simulink model "aa_IOT"  (R2024b)
settings: Solver=VariableStepAuto  StartTime=0.0  StopTime=0.20  RelTol=1e-3
undefined symbols (not defined in the file): Acid, Ion, Lead, Lithium, sigbuilder_block
libraries: spsBreakerLib x120, spsBatteryLib x72, spsSeriesRLCBranchLib x47, spsVoltageMeasurementLib x33, spsIdealSwitchLib x19, spsDiodeLib x10, spsCurrentMeasurementLib x8, spsThyristorLib x6, sldrtlib x4, spsACVoltageSourceLib x3, spsIGBTLib x2, spsPVArrayLib x1
(part 1 of 7)
settings Model: SimulationMode=accelerator  Creator=Jatay  LastModifiedBy=Jatay

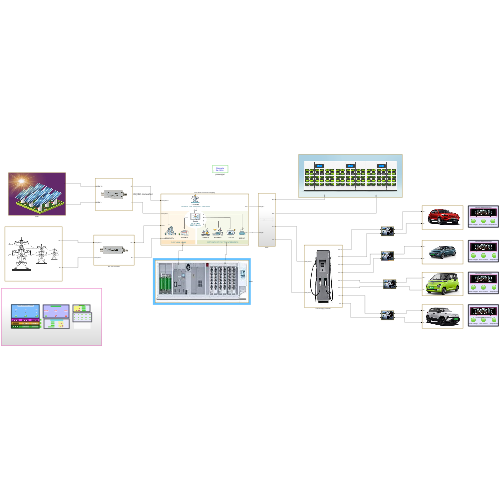
[thumbnail: Simulink's stored preview of the top-level diagram]
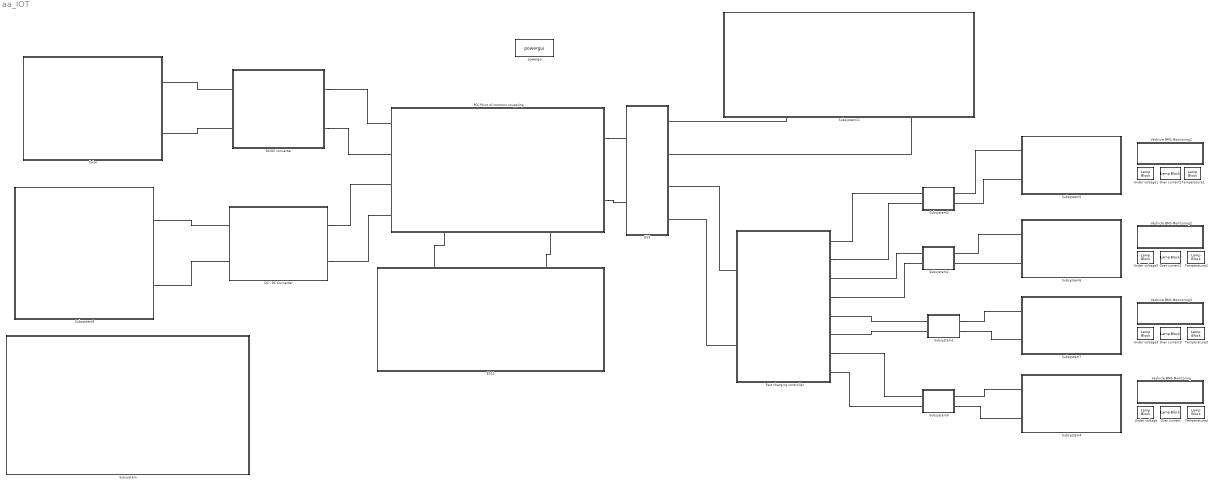
== system aa_IOT ==
  DC - DC Converter : Subsystem
      mask Display: image('cc_converter.png');
  DC/DC converter : Subsystem
      mask Display: image('cc_converter.png');
  ESS : Subsystem
  ESS1 : Subsystem
      mask Display: image('ess.jpeg');
  Fast charging controller : Subsystem
      mask Display: image('FC.jpeg');
  Over current{,1..3} (4 alike) : LampBlock  LabelPosition=Hide
  PCC Point of common couppling : Subsystem
      settings: PortSchema="{\"entries\":[{\"content\":{\"sides\":[{\"content\":{\"connectorIds\":[\"LConn1\",\"LConn2\",\"LConn3\",\"LConn4\"]},\"type\":\"ConnectorPlacement.EquallySpacedRectSide\",\"uuid\":\"0b8ed45c-57e4-41e0-bfb2-9585222a0f80\"},{\"content\":{\"connectorIds\":[\"RConn1\",\"RConn2\"],\"side\":\"RIGHT\"},\"type\":\"ConnectorPlacement.EquallySpacedRectSide\",\"uuid\":\"94498682-9e53-424b-ae3f-72f463f0ef3d\"},{\"content\":{\"side\":\"TOP\"},\"type\":\"ConnectorPlacement.EquallySpacedRectSide\",\"uuid\":\"67a2b653-7e16-402f-9cd2-3c5333b5ea45\"},{\"content\":{\"connectorIds\":[\"RConn3\",\"RConn4\"],\"side\":\"BOTTOM\"},\"type\":\"ConnectorPlacement.EquallySpacedRectSide\",\"uuid\":\"cc71de87-45eb-4874-8a05-0c8232189766\"}]},\"type\":\"ConnectorPlacement.EquallySpacedConnector\",\"uuid\":\"bd8a6289-7e4b-491d-b567-63bc7d53a2fa\"}],\"packageUris\":[\"http://schema.mathworks.com/mf0/Connector/R2020b\"],\"version\":\"1.0\"}"
      mask Display: image('pcc.png');
  Solar : Subsystem
      mask Display: image('Solar-Power-Plant-1024x536.jpg');
  Subsystem : Subsystem
  Subsystem1 : Subsystem
      mask Display: image('plugin.jpeg');
  Subsystem11 : Subsystem
      mask Display: image('swapping.webp');
  Subsystem2 : Subsystem
      mask Display: image('plugin.jpeg');
  Subsystem3 : Subsystem
      mask Display: image('plugin.jpeg');
  Subsystem4 : Subsystem
      mask Display: image('ev_4.webp');
  Subsystem5 : Subsystem
      mask Display: image('ev_3.webp');
  Subsystem6 : Subsystem
      mask Display: image('ev_2.jpg');
  Subsystem7 : Subsystem
      mask Display: image('ev-1.jpeg');
  Subsystem8 : Subsystem
      mask Display: image('grid.png');
  Subsystem9 : Subsystem
      mask Display: image('plugin.jpeg');
  Temperature{1..4} (4 alike) : LampBlock  LabelPosition=Hide
  Under voltage{,1..3} (4 alike) : LampBlock  LabelPosition=Hide
  Vechicle BMS Monitoring : Subsystem
      mask Display: image('Dash_board.jpeg');
  Vechicle BMS Monitoring1 : Subsystem
      mask Display: image('Dash_board.jpeg');
  Vechicle BMS Monitoring2 : Subsystem
      mask Display: image('Dash_board.jpeg');
  Vechicle BMS Monitoring3 : Subsystem
      mask Display: image('Dash_board.jpeg');
  powergui : sps_lib/powergui  Priority=1  SimulationMode=Discrete  SampleTime=5e-6  frequency=60  Iterations=50  frequencyindice=0  Pbase=100e6  ErrMax=1e-4  UnitsV=kV  UnitsW=MW  buscounter=0  FunctionMessages=off  echomessages=off  EnableUseOfTLC=off  CurrentSourceSwitches=off  DisableSnubberDevices=off  DisableRonSwitches=off  DisableVfSwitches=off  DisplayEquations=off  AutomaticDiscreteSolvers=off  SolverType=Tustin  Interpol=off  ExternalGateDelay=off  methode=off  Ts=0  x0status=blocks  SPID=off  SwTol=0  HookPort=off  NonlinearTolerance=1e-4  nMaxIteration=100  ContinueOnMaxIteration=off  RestoreLinks=warning  ResistiveCurrentMeasurement=off  Frange=[0:2:500]  Ylog=off  Xlog=on  ShowGrid=off  save=off  variable=ZData  structure=0  ZoomFFT=off  StartTime=0.0  cycles=1  DisplayStyle=1  fundamental=60  FreqAxis=off  MaxFrequency=1000  frequencyindicesteady=1  RmsSteady=1  display=off
  connections:
  DC/DC converter/LConn2 -- Solar/RConn2
  DC/DC converter/LConn1 -- Solar/RConn1
  PCC Point of common couppling/RConn2 -- ESS/LConn2
  Subsystem8/RConn2 -- DC - DC Converter/LConn2
  Subsystem8/RConn1 -- DC - DC Converter/LConn1
  PCC Point of common couppling/RConn1 -- ESS/LConn1
  DC/DC converter/RConn1 -- PCC Point of common couppling/LConn1
  DC/DC converter/RConn2 -- PCC Point of common couppling/LConn2
  DC - DC Converter/RConn1 -- PCC Point of common couppling/LConn3
  DC - DC Converter/RConn2 -- PCC Point of common couppling/LConn4
  Subsystem11/LConn1 -- ESS/RConn1
  Subsystem11/LConn2 -- ESS/RConn2
  Subsystem9/LConn2 -- Fast charging controller/RConn1
  Fast charging controller/RConn5 -- Subsystem2/LConn2
  Fast charging controller/RConn2 -- Subsystem9/LConn1
  Subsystem1/LConn2 -- Fast charging controller/RConn3
  Fast charging controller/RConn7 -- Subsystem3/LConn2
  Subsystem3/LConn1 -- Fast charging controller/RConn8
  Subsystem2/LConn1 -- Fast charging controller/RConn6
  Subsystem1/LConn1 -- Fast charging controller/RConn4
  ESS1/RConn1 -- PCC Point of common couppling/RConn3
  ESS1/RConn2 -- PCC Point of common couppling/RConn4
  Fast charging controller/LConn2 -- ESS/RConn3
  Fast charging controller/LConn1 -- ESS/RConn4
  Subsystem5/LConn1 -- Subsystem3/RConn1
  Subsystem5/LConn2 -- Subsystem3/RConn2
  Subsystem6/LConn1 -- Subsystem2/RConn1
  Subsystem6/LConn2 -- Subsystem2/RConn2
  Subsystem1/RConn1 -- Subsystem7/LConn1
  Subsystem1/RConn2 -- Subsystem7/LConn2
  Subsystem4/LConn1 -- Subsystem9/RConn1
  Subsystem9/RConn2 -- Subsystem4/LConn2

== system aa_IOT/DC - DC Converter ==
  Diode : spsDiodeLib/Diode  Ron=0.001  Lon=0  Vf=1.1  IC=0  UseSnubber=off  Rs=500  Cs=250e-9  Measurements=off
  Diode2 : spsDiodeLib/Diode  Ron=0.001  Lon=0  Vf=0.7  IC=0  UseSnubber=off  Rs=500  Cs=250e-9  Measurements=off
  Display1 : Display
  Display2 : Display
  RL : spsSeriesRLCBranchLib/Series RLC Branch  LConnTagsString=__new0  RConnTagsString=__new0  BranchType=RL  Resistance=0.05  Inductance=470e-6  SetiL0=off  InitialCurrent=0  Capacitance=1e-6  Setx0=off  InitialVoltage=0  Measurements=None
  Voltage Measurement1 : spsVoltageMeasurementLib/Voltage Measurement  PhasorSimulation=off  OutputType=Complex  PSBequivalent=0
  Voltage Measurement2 : spsVoltageMeasurementLib/Voltage Measurement  PhasorSimulation=off  OutputType=Complex  PSBequivalent=0
  DC + : PMIOPort  Side=Right
  solar panel + : PMIOPort  Port=2  Side=Left
  solar panel - : PMIOPort  Port=3  Side=Left
  DC - : PMIOPort  Port=4  Side=Right
  wires:
  Voltage Measurement1/1 -> Display1/1
  Voltage Measurement2/1 -> Display2/1
  connections:
  solar panel +/RConn1 -- Voltage Measurement1/LConn1 -- DC +/RConn1 -- Voltage Measurement2/LConn1 -- Diode/RConn1 -- Diode2/LConn1
  Diode2/RConn1 -- RL/LConn1
  Diode/LConn1 -- RL/RConn1
  DC -/RConn1 -- Voltage Measurement1/LConn2 -- solar panel -/RConn1 -- Voltage Measurement2/LConn2

== system aa_IOT/DC//DC converter ==
  Battery : spsBatteryLib/Battery  BatType=Lead-Acid  NomV=400  NomQ=100  SOC=100  Batt_Tr=30  PresetModel=on  MaxQ=104.1667  MinV=300  FullV=435.5263  Dis_rate=20  R=0.04  Normal_OP=31.0278  expZone="[407.2368     0.3333333]"
  DC - DC Converter : Subsystem
  DC bus : Subsystem
  Display : Display
  Voltage Measurement : spsVoltageMeasurementLib/Voltage Measurement  PhasorSimulation=off  OutputType=Complex  PSBequivalent=0
  Voltage Measurement2 : spsVoltageMeasurementLib/Voltage Measurement  PhasorSimulation=off  OutputType=Complex  PSBequivalent=0
  solar + : PMIOPort  Side=Left
  solar - : PMIOPort  Port=2  Side=Left
  + : PMIOPort  Port=3  Side=Right
  - : PMIOPort  Port=4  Side=Right
  tag scope: solar_controller=global
  wires:
  Voltage Measurement2/1 -> [solar_controller]
  Voltage Measurement/1 -> Display/1
  connections:
  DC - DC Converter/RConn1 -- DC bus/LConn1
  solar +/RConn1 -- DC - DC Converter/LConn1 -- Voltage Measurement2/LConn1
  DC - DC Converter/LConn2 -- Voltage Measurement2/LConn2 -- solar -/RConn1
  DC - DC Converter/RConn2 -- DC bus/LConn2
  -/RConn1 -- Battery/LConn2 -- DC bus/RConn2 -- Voltage Measurement/LConn2
  Voltage Measurement/LConn1 -- Battery/LConn1 -- DC bus/RConn1 -- +/RConn1

== system aa_IOT/ESS ==
  Display : Display
  Voltage Measurement : spsVoltageMeasurementLib/Voltage Measurement  PhasorSimulation=off  OutputType=Complex  PSBequivalent=0
  Charger + : PMIOPort  Side=Left
  Charger - : PMIOPort  Port=2  Side=Left
  BS + : PMIOPort  Port=3  Side=Right
  BS - : PMIOPort  Port=4  Side=Right
  FC + : PMIOPort  Port=5  Side=Right
  FC - : PMIOPort  Port=6  Side=Right
  wires:
  Voltage Measurement/1 -> Display/1
  connections:
  FC -/RConn1 -- Voltage Measurement/LConn2 -- Charger -/RConn1 -- BS -/RConn1
  Charger +/RConn1 -- Voltage Measurement/LConn1 -- FC +/RConn1 -- BS +/RConn1

== system aa_IOT/ESS1 ==
  DC - DC Converter : Subsystem
      mask Display: image('cc_converter.png');
  Display1 : Display
  Subsystem : Subsystem
  Voltage Measurement1 : spsVoltageMeasurementLib/Voltage Measurement  PhasorSimulation=off  OutputType=Complex  PSBequivalent=0
  ESS ++ : PMIOPort  Side=Right
  ESS -- : PMIOPort  Port=2  Side=Right
  wires:
  Voltage Measurement1/1 -> Display1/1
  connections:
  Subsystem/LConn1 -- Voltage Measurement1/LConn1 -- DC - DC Converter/LConn1
  Subsystem/LConn2 -- Voltage Measurement1/LConn2 -- DC - DC Converter/LConn2
  ESS ++/RConn1 -- DC - DC Converter/RConn1
  ESS --/RConn1 -- DC - DC Converter/RConn2

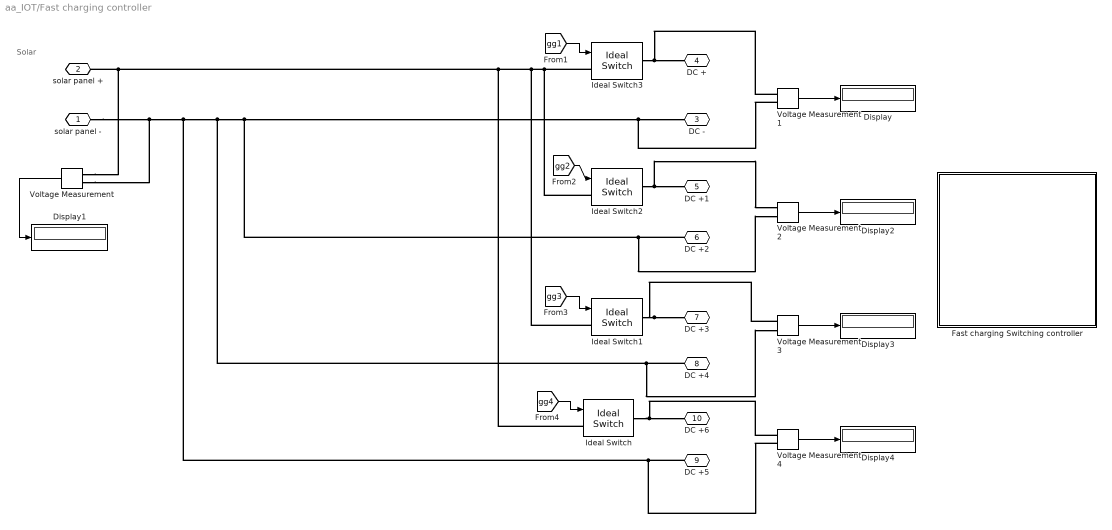
== system aa_IOT/Fast charging controller ==
  note: Solar
  Display{,1..4} (5 alike) : Display
  Fast charging Switching controller : Subsystem
  Ideal Switch{,1..3} (4 alike) : spsIdealSwitchLib/Ideal Switch  Ron=0.001  Lon=0  IC=0  Rs=1e5  Cs=inf  Measurements=off
  Voltage Measurement{,1..4} (5 alike) : spsVoltageMeasurementLib/Voltage Measurement  PhasorSimulation=off  OutputType=Complex  PSBequivalent=0
  solar panel - : PMIOPort  Side=Left
  solar panel + : PMIOPort  Port=2  Side=Left
  DC - : PMIOPort  Port=3  Side=Right
  DC + : PMIOPort  Port=4  Side=Right
  DC +1 : PMIOPort  Port=5  Side=Right
  DC +2 : PMIOPort  Port=6  Side=Right
  DC +3 : PMIOPort  Port=7  Side=Right
  DC +4 : PMIOPort  Port=8  Side=Right
  DC +5 : PMIOPort  Port=9  Side=Right
  DC +6 : PMIOPort  Port=10  Side=Right
  wires:
  [gg1] -> Ideal Switch3/1
  [gg2] -> Ideal Switch2/1
  [gg3] -> Ideal Switch1/1
  [gg4] -> Ideal Switch/1
  Voltage Measurement/1 -> Display1/1
  Voltage Measurement1/1 -> Display/1
  Voltage Measurement2/1 -> Display2/1
  Voltage Measurement3/1 -> Display3/1
  Voltage Measurement4/1 -> Display4/1
  connections:
  Ideal Switch3/LConn1 -- Ideal Switch2/LConn1 -- Ideal Switch1/LConn1 -- Ideal Switch/LConn1 -- Voltage Measurement/LConn1 -- solar panel +/RConn1
  solar panel -/RConn1 -- Voltage Measurement/LConn2 -- Voltage Measurement4/LConn2 -- DC +5/RConn1 -- Voltage Measurement3/LConn2 -- DC +4/RConn1 -- Voltage Measurement2/LConn2 -- DC +2/RConn1 -- Voltage Measurement1/LConn2 -- DC -/RConn1
  Ideal Switch3/RConn1 -- Voltage Measurement1/LConn1 -- DC +/RConn1
  Ideal Switch1/RConn1 -- DC +3/RConn1 -- Voltage Measurement3/LConn1
  Ideal Switch/RConn1 -- DC +6/RConn1 -- Voltage Measurement4/LConn1
  Ideal Switch2/RConn1 -- Voltage Measurement2/LConn1 -- DC +1/RConn1

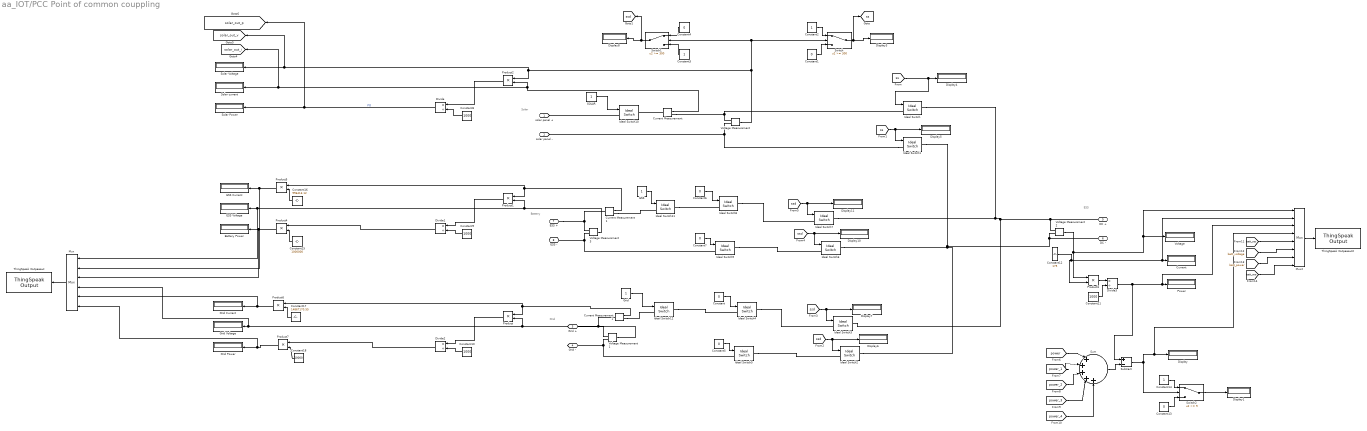
== system aa_IOT/PCC Point of common couppling ==
  note: ESS
  note: Grid
  note: Solar
  note: Battery
  Battery Power : Display
  Constant{,1,4..7,13} (7 alike) : Constant  Value=0
  Constant{8..11} (4 alike) : Constant  Value=1000
  Constant12 : Constant  Value=175
  Constant14 : Constant
  Constant15 : Constant  Value=1000000
  Constant16 : Constant  Value=996413.12
  Constant17 : Constant  Value=14867170.55
  Constant18 : Constant  Value=10000
  Constant2 : Constant
  Constant3 : Constant
  Current : Display
  Current Measurement : spsCurrentMeasurementLib/Current Measurement  PhasorSimulation=off  OutputType=Complex  PSBequivalent=0
  Current Measurement1 : spsCurrentMeasurementLib/Current Measurement  PhasorSimulation=off  OutputType=Complex  PSBequivalent=0
  Current Measurement2 : spsCurrentMeasurementLib/Current Measurement  PhasorSimulation=off  OutputType=Complex  PSBequivalent=0
  Display{,1,3..8,10..11} (10 alike) : Display
  Divide{,1..3} (4 alike) : Product  Inputs=*/
  ESS : Constant
  "ESS Current " : Display
  ESS Voltage : Display
  Grid : Constant
  Grid Current : Display
      settings: Format=short_e
  Grid Power : Display
  Grid Voltage : Display
  Ideal Switch{,1..3,6..7,10..12} (9 alike) : spsIdealSwitchLib/Ideal Switch  Ron=0.001  Lon=0  IC=0  Rs=1e5  Cs=inf  Measurements=off
  Ideal Switch{4..5,8..9} (4 alike) : spsIdealSwitchLib/Ideal Switch  Ron=0.01  Lon=0  IC=0  Rs=1e5  Cs=inf  Measurements=off
  Mux : Mux  Inputs=6
  Mux2 : Mux  Inputs=8
  Power : Display
  Product{,1..7} (8 alike) : Product
  SOLAR : Constant
  Solar Power : Display
  Solar Voltage : Display
  Solar current : Display
  Subtract : Sum  Inputs=+-
  Sum : Sum  Inputs=|+++++
  Switch : Switch  Threshold=300  SaturateOnIntegerOverflow=off  InputSameDT=off
  Switch1 : Switch  Threshold=300  SaturateOnIntegerOverflow=off  InputSameDT=off
  Switch2 : Switch  Threshold=9  SaturateOnIntegerOverflow=off  InputSameDT=off
  ThingSpeak Outpaaaut : sldrtlib/Internet of Things/ThingSpeak Output  DrvAddress=2749674  DrvOptions=[1 20 66 79 84 51 68 69 56 84 69 80 84 72 55 77 55 70 97 112 105 46 116 104 105 110 103 115 112 101 97 107 46 99 111 109 0 0 0 0 0 0 0 0 0 0 0 0 0 0 0 0 0 0 0 0 0 0 0 0 0 0 0 0 0 0 0 0 0 0 0 0 0 0 0 0 0 0 0 0 0 0 0 0 0 0 0 0 0 0 0 0 0 0 0 0 0 0 0 0 0 0 0 0 0 0 0 0 0 0 0 0 0 0 0 0 0 0 0 0 0 0 0 0 0 0 0 0 0 0 0 0 0 0 0 0 0 0 0 0 0 0 0 0 0 0 0 0 0 0 0 0 0 0 0 0 0 0 0 0 0 0 0 0 0 0 0 0 0 0 0 0 0 0 0 0 0 0 0 0 0 0 0 0 0 0 0 0 0 0 0 0 0 0 0 0 0 0 0 0 0 0 0 0 0 0 0 0 0 0 0 0 0 0 0 0 0 0 0 0 0 0 0 0 0 0 0 0 0 0 0 0 0 0 0 0 0 0 0 0 0 0 0 0 0 0 0 0 0 0 0 0 0 0 0 0]  SampleTime=0.1  MaxMissedTicks=1000000000000000000000000000000  ShowMissedTicks=off  YieldWhenWaiting=off  ChannelFields=[1 2 3 4 5 6]  OptParam=0  InitialValue=[]  FinalValue=[]
  ThingSpeak Outpaaaut2 : sldrtlib/Internet of Things/ThingSpeak Output  DrvAddress=2750723  DrvOptions=[1 20 68 52 66 89 74 56 54 84 81 57 48 90 75 88 50 78 97 112 105 46 116 104 105 110 103 115 112 101 97 107 46 99 111 109 0 0 0 0 0 0 0 0 0 0 0 0 0 0 0 0 0 0 0 0 0 0 0 0 0 0 0 0 0 0 0 0 0 0 0 0 0 0 0 0 0 0 0 0 0 0 0 0 0 0 0 0 0 0 0 0 0 0 0 0 0 0 0 0 0 0 0 0 0 0 0 0 0 0 0 0 0 0 0 0 0 0 0 0 0 0 0 0 0 0 0 0 0 0 0 0 0 0 0 0 0 0 0 0 0 0 0 0 0 0 0 0 0 0 0 0 0 0 0 0 0 0 0 0 0 0 0 0 0 0 0 0 0 0 0 0 0 0 0 0 0 0 0 0 0 0 0 0 0 0 0 0 0 0 0 0 0 0 0 0 0 0 0 0 0 0 0 0 0 0 0 0 0 0 0 0 0 0 0 0 0 0 0 0 0 0 0 0 0 0 0 0 0 0 0 0 0 0 0 0 0 0 0 0 0 0 0 0 0 0 0 0 0 0 0 0 0 0 0 0]  SampleTime=0.1  MaxMissedTicks=1000000000000000000000000000000  ShowMissedTicks=off  YieldWhenWaiting=off  ChannelFields=[1 2 3 4 5 6 7 8]  OptParam=0  InitialValue=[]  FinalValue=[]
  Voltage : Display
  Voltage Measurement{,1..3} (4 alike) : spsVoltageMeasurementLib/Voltage Measurement  PhasorSimulation=off  OutputType=Complex  PSBequivalent=0
  solar panel + : PMIOPort  Side=Left
  solar panel - : PMIOPort  Port=2  Side=Left
  Grid + : PMIOPort  Port=3  Side=Left
  Grid - : PMIOPort  Port=4  Side=Left
  DC + : PMIOPort  Port=5  Side=Right
  DC - : PMIOPort  Port=6  Side=Right
  ESS + : PMIOPort  Port=7  Side=Right
  ESS - : PMIOPort  Port=8  Side=Right
  tag scope: solar_out_i=global, solar_out_p=global, solar_out_v=global, ss=global, ssd=global
  wires:
  Voltage Measurement1/1 -> Product/2, Mux/4, Grid Voltage/1
  Voltage Measurement2/1 -> Mux2/1, Voltage/1, Product3/1
  Switch/1 -> Display3/1, [ss]
  Constant2/1 -> Switch/1
  Constant1/1 -> Switch/3
  [ss] -> Ideal Switch/1, Display4/1
  [ss] -> Ideal Switch1/1, Display5/1
  [ssd] -> Ideal Switch2/1, Display6/1
  [ssd] -> Ideal Switch3/1, Display7/1
  Constant3/1 -> Switch1/3
  Voltage Measurement/1 -> Switch/2, Switch1/2, Product2/1, [solar_out_v], Solar Voltage/1
  Constant4/1 -> Switch1/1
  Switch1/1 -> Display8/1, [ssd]
  Constant/1 -> Ideal Switch4/1
  Constant5/1 -> Ideal Switch5/1
  [ssd] -> Ideal Switch7/1, Display11/1
  Constant7/1 -> Ideal Switch9/1
  Constant6/1 -> Ideal Switch8/1
  [ssd] -> Ideal Switch6/1, Display10/1
  Voltage Measurement3/1 -> Product1/2, Mux/1, ESS Voltage/1
  SOLAR/1 -> Ideal Switch10/1
  ESS/1 -> Ideal Switch11/1
  Grid/1 -> Ideal Switch12/1
  Product2/1 -> Divide/1
  Constant8/1 -> Divide/2
  Product1/1 -> Divide1/1
  Constant9/1 -> Divide1/2
  Product/1 -> Divide2/1
  Constant10/1 -> Divide2/2
  Constant11/1 -> Divide3/2
  Constant12/1 -> Product3/2, Mux2/2, Current/1
  Product3/1 -> Divide3/1
  Divide3/1 -> Subtract/1, Mux2/3, Power/1
  Sum/1 -> Subtract/2
  Constant13/1 -> Switch2/3
  Subtract/1 -> Mux2/4, Display/1, Switch2/2
  Switch2/1 -> Display1/1
  Constant14/1 -> Switch2/1
  [power] -> Sum/1
  [power_1] -> Sum/2
  [power_2] -> Sum/3
  [power_4] -> Sum/5
  [power_3] -> Sum/4
  Divide/1 -> Solar Power/1, [solar_out_p]  "PO"
  Current Measurement/1 -> Product2/2, [solar_out_i], Solar current/1
  Mux/1 -> ThingSpeak Outpaaaut/1
  Product4/1 -> Mux/3, Battery Power/1
  Divide1/1 -> Product4/1
  Constant15/1 -> Product4/2
  Constant16/1 -> Product5/2
  Current Measurement1/1 -> Product1/1, Product5/1
  Product5/1 -> Mux/2, "ESS Current "/1
  Constant17/1 -> Product6/2
  Current Measurement2/1 -> Product6/1, Product/1
  Product6/1 -> Mux/5, Grid Current/1
  Constant18/1 -> Product7/2
  Divide2/1 -> Product7/1
  Product7/1 -> Mux/6, Grid Power/1
  Mux2/1 -> ThingSpeak Outpaaaut2/1
  [batt_soc] -> Mux2/5
  [batt_voltage] -> Mux2/6
  [batt_power] -> Mux2/7
  [batt_ava] -> Mux2/8
  connections:
  Ideal Switch1/RConn1 -- DC -/RConn1 -- Voltage Measurement2/LConn2 -- Ideal Switch2/RConn1 -- Ideal Switch6/RConn1
  Voltage Measurement/LConn1 -- Current Measurement/RConn1 -- Ideal Switch/LConn1
  Voltage Measurement1/LConn2 -- Ideal Switch5/LConn1 -- Grid -/RConn1
  Grid +/RConn1 -- Voltage Measurement1/LConn1 -- Current Measurement2/LConn1
  Ideal Switch4/RConn1 -- Ideal Switch3/LConn1
  Ideal Switch3/RConn1 -- Ideal Switch7/RConn1 -- Ideal Switch/RConn1 -- Voltage Measurement2/LConn1 -- DC +/RConn1
  Ideal Switch1/LConn1 -- Voltage Measurement/LConn2 -- solar panel -/RConn1
  Ideal Switch5/RConn1 -- Ideal Switch2/LConn1
  ESS +/RConn1 -- Current Measurement1/LConn1 -- Voltage Measurement3/LConn1
  ESS -/RConn1 -- Voltage Measurement3/LConn2 -- Ideal Switch9/LConn1
  Ideal Switch8/RConn1 -- Ideal Switch7/LConn1
  Ideal Switch9/RConn1 -- Ideal Switch6/LConn1
  Ideal Switch10/LConn1 -- solar panel +/RConn1
  Ideal Switch11/RConn1 -- Ideal Switch8/LConn1
  Ideal Switch12/RConn1 -- Ideal Switch4/LConn1
  Current Measurement/LConn1 -- Ideal Switch10/RConn1
  Current Measurement1/RConn1 -- Ideal Switch11/LConn1
  Current Measurement2/RConn1 -- Ideal Switch12/LConn1

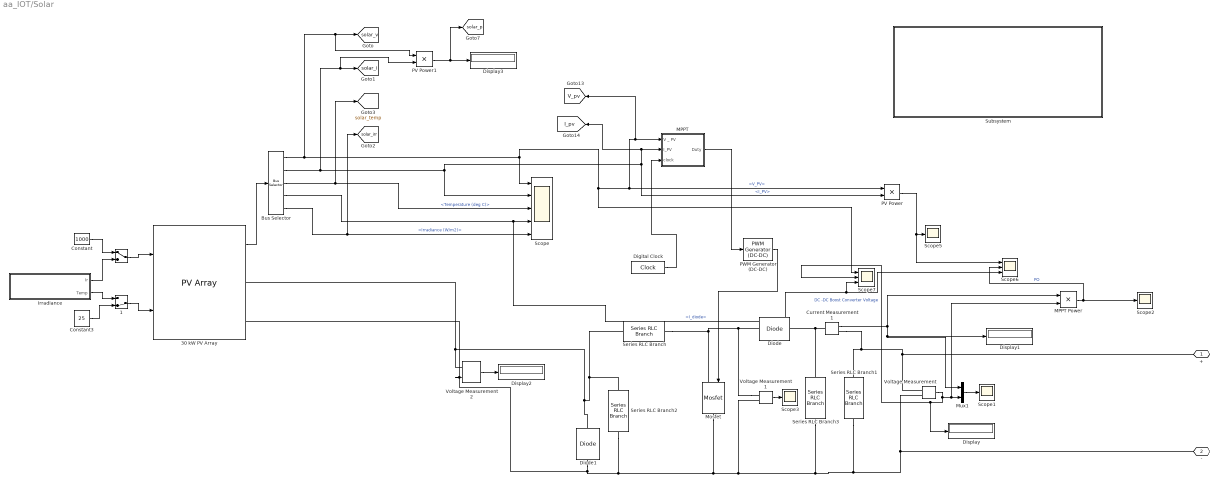
== system aa_IOT/Solar ==
  "      " : ManualSwitch
  "      1" : ManualSwitch  CurrentSetting=0
  30 kW PV Array : spsPVArrayLib/PV Array  Npar=15  Nser=10  PlotType=array @ 1000 W/m2 & specified temperatures  S_vec="[ 1000  500  100 ]"  Temp_C_vec="[ 45 25  ]"  ModuleName=User-defined  PlotWhenSelected=off  Pm=213.15  Ncell=60  Voc=48  Isc=7.84  Vm=29  Im=7.35  beta_Voc_pc=-0.36099  alpha_Isc_pc=0.102  beta_Voc=-0.17328  alpha_Isc=0.0079968  IL=8.2285  I0=2.9956e-10  nI=1.2955  Rsh=7353.5939  Rs=2.0228  RobustModel=off  RobustCellTemperature=25  BAL=on  Tc=1e-6  Tfilter=5e-5
  Bus Selector : BusSelector  OutputSignals=V_PV,I_PV,Temperature (deg C),I_diode,Irradiance (W/m2)
  Constant : Constant  Value=1000
  Constant3 : Constant  Value=25
  Current Measurement1 : spsCurrentMeasurementLib/Current Measurement  PhasorSimulation=off  OutputType=Complex  PSBequivalent=0
  Digital Clock : DigitalClock  SampleTime=0.001
  Diode : spsDiodeLib/Diode  Ron=0.5  Lon=0  Vf=0.7  IC=0  UseSnubber=0  Rs=1e5  Cs=250e-9  Measurements=off
  Diode1 : spsDiodeLib/Diode  Ron=0.5  Lon=0  Vf=0.7  IC=0  UseSnubber=0  Rs=1e5  Cs=250e-9  Measurements=off
  Display{,1..3} (4 alike) : Display
  "Irradiance " : Subsystem  Tag=STV Subsys  LoadFcn=sigbuilder_block('load');  StartFcn=sigbuilder_block('start');  StopFcn=sigbuilder_block('stop');  ClipboardFcn=sigbuilder_block('clipboard');  mask(Sigbuilder block){tuvar=[0:10]}
      mask help: Sigbuilder GUI
      mask init:
      | if ~strcmp(get_param(bdroot(gcbh),'SimulationStatus'),'stopped') tuvar = sigbuilder_block('maskInit'); end
      settings: CopyFcn=sigbuilder_block('copy');  DeleteFcn=sigbuilder_block('delete');  ModelCloseFcn=sigbuilder_block('modelClose');  PreSaveFcn=sigbuilder_block('preSave');  PauseFcn=sigbuilder_block('pause')  ContinueFcn=sigbuilder_block('continue')  NameChangeFcn=sigbuilder_block('namechange');  OpenFcn=sigbuilder_block('open',[5.4 30 1141.2 507.6 ]);  CloseFcn=sigbuilder_block('close');
      mask Display: plot(0, 0, 100, 100,[2, 2, 32, 32, 2], [68, 8, 8, 68, 68],[32, 2], [38, 38], [32, 19, 2],[53, 60, 44], [32, 17, 17, 2],[16, 16, 31, 31]);txt = getActiveGroup(gcbh);text(2, 100, txt,'verticalAlignment', 'top');
  MPPT : Subsystem
  MPPT Power : Product
  Mosfet : spsMosfetLib/Mosfet  Ron=0.1  Lon=0  Rd=0.01  Vfd=0.7  IC=0  Rs=1e5  Cs=inf  Measurements=off
  Mux1 : Mux  Inputs=2
  PV Power : Product
  PV Power1 : Product
  PWM Generator (DC-DC) : spsPWMGeneratorDCDCLib/PWM Generator (DC-DC)  Fsw=1500  Ts=0
  Scope : Scope  NumInputPorts=5
  Scope{1..3,5} (4 alike) : Scope
  Scope6 : Scope  NumInputPorts=3
  Scope7 : Scope  NumInputPorts=3
  Series RLC Branch : spsSeriesRLCBranchLib/Series RLC Branch  LConnTagsString=__new0  RConnTagsString=__new0  BranchType=L  Resistance=0.001  Inductance=0.4e-1  SetiL0=off  InitialCurrent=0  Capacitance=1e-6  Setx0=off  InitialVoltage=0  Measurements=None
  Series RLC Branch1 : spsSeriesRLCBranchLib/Series RLC Branch  LConnTagsString=__new0  RConnTagsString=__new0  BranchType=R  Resistance=11  Inductance=0.1  SetiL0=off  InitialCurrent=0  Capacitance=100e-6  Setx0=off  InitialVoltage=0  Measurements=None
  Series RLC Branch2 : spsSeriesRLCBranchLib/Series RLC Branch  LConnTagsString=__new0  RConnTagsString=__new0  BranchType=C  Resistance=6  Inductance=0.1  SetiL0=off  InitialCurrent=0  Capacitance=700e-5  Setx0=off  InitialVoltage=0  Measurements=None
  Series RLC Branch3 : spsSeriesRLCBranchLib/Series RLC Branch  LConnTagsString=__new0  RConnTagsString=__new0  BranchType=C  Resistance=6  Inductance=0.1  SetiL0=off  InitialCurrent=0  Capacitance=1000e-5  Setx0=off  InitialVoltage=0  Measurements=None
  Subsystem : Subsystem
  Voltage Measurement : spsVoltageMeasurementLib/Voltage Measurement  PhasorSimulation=off  OutputType=Complex  PSBequivalent=0
  Voltage Measurement1 : spsVoltageMeasurementLib/Voltage Measurement  PhasorSimulation=off  OutputType=Complex  PSBequivalent=0
  Voltage Measurement2 : spsVoltageMeasurementLib/Voltage Measurement  PhasorSimulation=off  OutputType=Complex  PSBequivalent=0
  + : PMIOPort  Side=Right
  - : PMIOPort  Port=2  Side=Right
  tag scope: I_pv=global, V_pv=global, solar_i=global, solar_irr=global, solar_p=global, solar_temp=global, solar_v=global
  wires:
  Voltage Measurement/1 -> MPPT Power/2, Mux1/2, Display/1, Scope7/2  "DC -DC Boost Converter Voltage"
  PWM Generator (DC-DC)/1 -> Mosfet/1
  Mux1/1 -> Scope1/1
  MPPT Power/1 -> Scope6/2, Scope2/1  "PO"
  Current Measurement1/1 -> MPPT Power/1, Display1/1, Mux1/1
  Voltage Measurement1/1 -> Scope3/1
  Bus Selector/3 -> [solar_temp], Scope/3  "<Temperature (deg C)>"
  Bus Selector/4 -> Scope6/3, Scope7/3, Scope/4  "<I_diode>"
  Digital Clock/1 -> MPPT/3(clock)
  MPPT/1(Duty) -> PWM Generator (DC-DC)/1
  PV Power/1 -> Scope6/1, Scope5/1
  "Irradiance "/2(Temp) -> "      1"/1
  Constant3/1 -> "      1"/2
  "Irradiance "/1(Ir) -> "      "/2
  Constant/1 -> "      "/1
  "      "/1 -> 30 kW PV Array/1
  "      1"/1 -> 30 kW PV Array/2
  Voltage Measurement2/1 -> Display2/1
  30 kW PV Array/1 -> Bus Selector/1
  Bus Selector/2 -> PV Power1/2, [solar_i], MPPT/2(I_PV), [I_pv], PV Power/2, Scope/2  "<I_PV>"
  Bus Selector/5 -> [solar_irr], Scope/5  "<Irradiance (W/m2)>"
  Bus Selector/1 -> PV Power1/1, [solar_v], Scope7/1, PV Power/1, [V_pv], MPPT/1("V _ PV "), Scope/1  "<V_PV>"
  PV Power1/1 -> [solar_p], Display3/1
  connections:
  Voltage Measurement/LConn2 -- Voltage Measurement2/LConn2 -- 30 kW PV Array/RConn2 -- Diode1/LConn1 -- Series RLC Branch2/RConn1 -- Mosfet/RConn1 -- Voltage Measurement1/LConn2 -- Series RLC Branch3/RConn1 -- Series RLC Branch1/RConn1 -- -/RConn1
  Current Measurement1/RConn1 -- Series RLC Branch1/LConn1 -- Voltage Measurement/LConn1 -- +/RConn1
  Diode/RConn1 -- Series RLC Branch3/LConn1 -- Current Measurement1/LConn1
  Voltage Measurement1/LConn1 -- Series RLC Branch/RConn1 -- Mosfet/LConn1 -- Diode/LConn1
  Series RLC Branch2/LConn1 -- Voltage Measurement2/LConn1 -- 30 kW PV Array/RConn1 -- Diode1/RConn1 -- Series RLC Branch/LConn1
